simulink model "min_state_observer"  (R2025b)
settings: Solver=VariableStepAuto  StartTime=0.0  StopTime=10  RelTol=1e-3
values from neighbouring files (symbols this model uses):
  A = [0 1 0 0 ; 0 -d/m m*g/M 0 ; 0 0 0 1; 0 -d/l*M (M+m)*g/(l*M) 0]    [CartPuller.m]    (also in Controller.m = [0 1 0 0; Ex12_4.m = [-5 1 0;0 -2 1;0 0 -1]; JacobCTP.m = [0 1 0 0; Observer_4state.m = [0 1; -k/m -c/m])
  A_hat = A_bb - Ke*A_ab    [Controller.m]    (also in min_state_observer.m)
  B = [0 1/M 0 1/(M*l)]'    [CartPuller.m]    (also in Controller.m = [0;1/m1;0;0]; Ex12_4.m = [0;0;1]; Observer_4state.m = [0; 1/m]; full_order_observer_smd.m = [0 0 0 1/m2]')
  B_hat = A_hat*Ke + A_ba - Ke*A_aa    [Controller.m]    (also in min_state_observer.m)
  C = eye(4)    [Controller.m]    (also in Ex12_4.m = [-1 1 0]; Observer_4state.m = [1 0]; full_order_observer_smd.m = [1 0 0 0]; full_state_observer.m = [1 0 0 0])
  C_hat = [zeros(1, 3) ... (first row only)    [Controller.m]    (also in min_state_observer.m)
  D_hat = [1 ... (first row only)    [Controller.m]    (also in min_state_observer.m)
  F_hat = B_b - Ke*B_a    [Controller.m]    (also in min_state_observer.m)
  Ke = place(A_bb', A_ab', p_o)'    [Controller.m]    (also in Observer_4state.m = place(A', C', p_o)'; full_order_observer_smd.m = place(A',C',p)'; min_state_observer.m; observer_E1.m = place(A', C', p_o)')
  x0 = [0;0;pi/3+0.1;0]    [CartPuller.m]    (also in CartPullerODE.m; Controller.m = [1; 0; -1; 0]; JacobCTP.m = [0;0;pi+.1;0]; Observer_4state.m = [-2 0 -10 -1])
  z0 = [2; 1.5; 1]    [Controller.m]    (also in min_state_observer.m)
settings Model: Creator=abhi  LastModifiedBy=Abhi

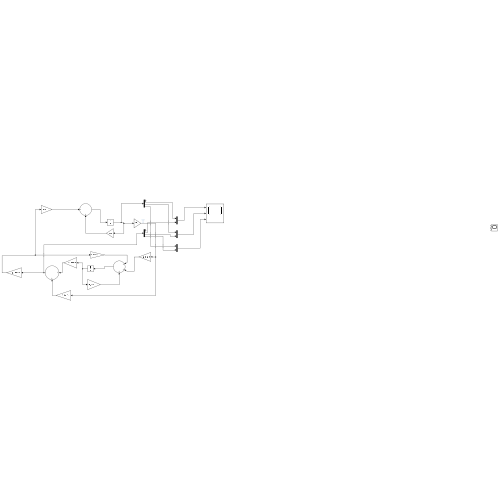
[thumbnail: Simulink's stored preview of the top-level diagram]
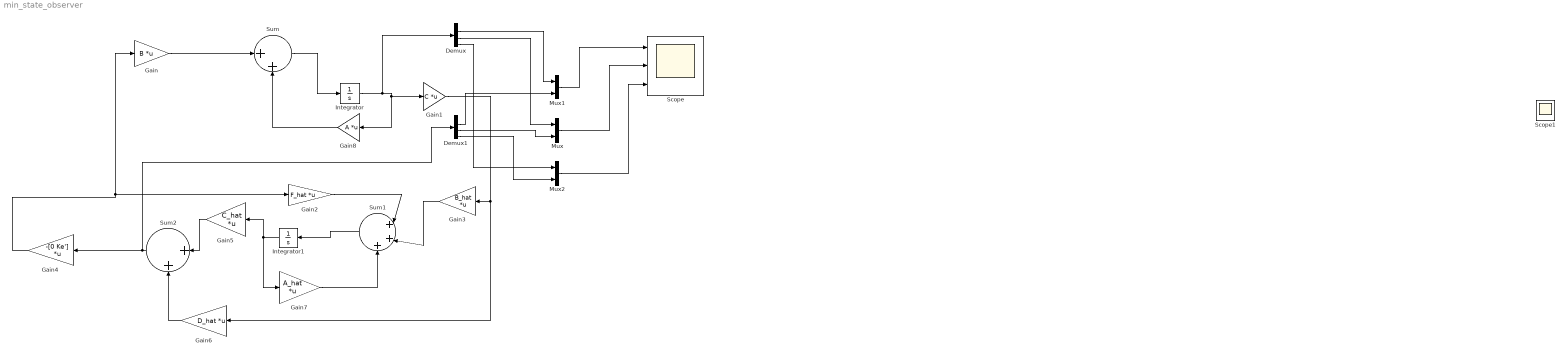
== system min_state_observer ==
  Demux : Demux
  Demux1 : Demux
  Gain : Gain  Gain=B  Multiplication=Matrix(K*u)
  Gain1 : Gain  Gain=C  Multiplication=Matrix(K*u)
  Gain2 : Gain  Gain=F_hat  Multiplication=Matrix(K*u)
  Gain3 : Gain  Gain=B_hat  Multiplication=Matrix(K*u)
  Gain4 : Gain  Gain=-[0 Ke']  Multiplication=Matrix(K*u)
  Gain5 : Gain  Gain=C_hat  Multiplication=Matrix(K*u)
  Gain6 : Gain  Gain=D_hat  Multiplication=Matrix(K*u)
  Gain7 : Gain  Gain=A_hat  Multiplication=Matrix(K*u)
  Gain8 : Gain  Gain=A  Multiplication=Matrix(K*u)
  Integrator : Integrator  InitialCondition=x0
  Integrator1 : Integrator  InitialCondition=z0
  Mux : Mux  Inputs=2
  Mux1 : Mux  Inputs=2
  Mux2 : Mux  Inputs=2
  Scope : Scope  NumInputPorts=3
      settings: ActiveDisplayYMinimum=-4.55722275159347  ActiveDisplayYMaximum=13.135987713140057
  Scope1 : Scope  NumInputPorts=2
      settings: ActiveDisplayYMinimum=-1.16819116268996  ActiveDisplayYMaximum=1.1667330676781473
  Sum : Sum  Inputs=|++
  Sum1 : Sum  Inputs=|+++
  Sum2 : Sum  Inputs=|++
  wires:
  Integrator/1 -> Demux/1, Gain8/1, Gain1/1
  Gain3/1 -> Sum1/2
  Gain2/1 -> Sum1/1
  Gain6/1 -> Sum2/2
  Gain5/1 -> Sum2/1
  Integrator1/1 -> Gain5/1, Gain7/1
  Gain7/1 -> Sum1/3
  Sum1/1 -> Integrator1/1
  Sum2/1 -> Gain4/1, Demux1/1
  Gain4/1 -> Gain/1, Gain2/1
  Gain1/1 -> Gain6/1, Gain3/1
  Sum/1 -> Integrator/1
  Gain8/1 -> Sum/2
  Gain/1 -> Sum/1
  Demux/3 -> Mux/1
  Demux1/3 -> Mux/2
  Demux/2 -> Mux1/1
  Demux1/2 -> Mux1/2
  Mux1/1 -> Scope/1
  Mux/1 -> Scope/2
  Demux/4 -> Mux2/1
  Demux1/4 -> Mux2/2
  Mux2/1 -> Scope/3
